simulink model "ActuatorControlLoop"  (R2019a)
settings: Solver=VariableStepAuto  StartTime=0.0  StopTime=10.0  RelTol=1e-3
undefined symbols (not defined in the file or in its folder): Kd, Ki, Kp
settings Model: DataDictionary=HeliSystemDD.sldd  OrderedModelArguments=off  Creator=bpotter  LastModifiedBy=bpotter
settings DataIOCC: ExternalInput=input  LoadExternalInput=on  SaveOutput=off  DSMLogging=off  SaveTime=off  ReturnWorkspaceOutputs=off  ReturnWorkspaceOutputsName=output
settings OptimizationCC: UseDivisionForNetSlopeComputation=on
settings ConfigComp: CovEnable=on  CovScope=ReferencedModels  CovIncludeTopModel=off  CovModelRefEnable=filtered  CovModelRefExcluded=FeedbackDelays,hydraulic_actuator,actuator

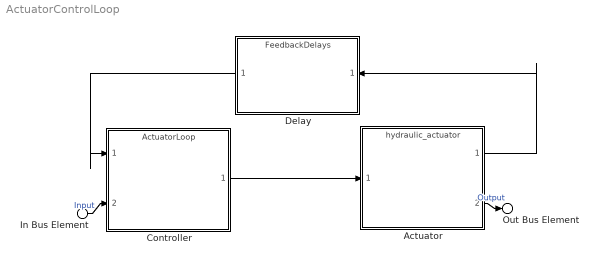
== system ActuatorControlLoop ==
  In Bus Element : Inport  PortName=Command
  Actuator : ModelReference  ModelNameDialog=hydraulic_actuator  SimulationMode=Normal  ModelReferenceVersion=1.109
      settings: PortSchema="{\"entries\":[{\"content\":{\"headerSize\":38,\"margin\":15,\"minimumSpacing\":25,\"sides\":[{\"content\":{\"connectorIds\":[\"In1\"]},\"type\":\"ConnectorPlacement.EquallySpacedRectSide\",\"uuid\":\"01d21f49-5e2a-4880-8609-7c706db9bae6\"},{\"content\":{\"connectorIds\":[\"Out1\",\"Out2\"],\"side\":\"RIGHT\"},\"type\":\"ConnectorPlacement.EquallySpacedRectSide\",\"uuid\":\"8cb49e98-f19c-489e-a3fb-070e8f82a61f\"},{\"content\":{\"connectorIds\":[],\"side\":\"TOP\"},\"type\":\"ConnectorPlacement.EquallySpacedRectSide\",\"uuid\":\"1c2cb19d-116b-4b67-8b19-5c9901225fc1\"}]},\"type\":\"ConnectorPlacement.EquallySpacedConnector\",\"uuid\":\"9f7d65ec-9623-4f05-bd53-df708bb30d55\"}],\"packageUris\":[\"http:\\/\\/schema.mathworks.com\\/mf0\\/Connector\\/19700101\"],\"version\":\"1.0\"}"
  Controller : ModelReference  ModelNameDialog=ActuatorLoop  ParameterArgumentNames=Kp,Kd,Ki  ParameterArgumentValues=0.135,-0.00134,0.00122  UsingDefaultArgumentValue=0,0,0  SimulationMode=Normal  ModelReferenceVersion=1.47
      settings: PortSchema="{\"entries\":[{\"content\":{\"headerSize\":38,\"margin\":15,\"minimumSpacing\":25,\"sides\":[{\"content\":{\"connectorIds\":[\"In1\",\"In2\"]},\"type\":\"ConnectorPlacement.EquallySpacedRectSide\",\"uuid\":\"01d21f49-5e2a-4880-8609-7c706db9bae6\"},{\"content\":{\"connectorIds\":[\"Out1\"],\"side\":\"RIGHT\"},\"type\":\"ConnectorPlacement.EquallySpacedRectSide\",\"uuid\":\"8cb49e98-f19c-489e-a3fb-070e8f82a61f\"},{\"content\":{\"connectorIds\":[],\"side\":\"TOP\"},\"type\":\"ConnectorPlacement.EquallySpacedRectSide\",\"uuid\":\"1c2cb19d-116b-4b67-8b19-5c9901225fc1\"}]},\"type\":\"ConnectorPlacement.EquallySpacedConnector\",\"uuid\":\"9f7d65ec-9623-4f05-bd53-df708bb30d55\"}],\"packageUris\":[\"http:\\/\\/schema.mathworks.com\\/mf0\\/Connector\\/19700101\"],\"version\":\"1.0\"}"
  Delay : ModelReference  ModelNameDialog=FeedbackDelays  SimulationMode=Normal  ModelReferenceVersion=1.165
      settings: PortSchema="{\"entries\":[{\"content\":{\"headerSize\":38,\"margin\":15,\"minimumSpacing\":25,\"sides\":[{\"content\":{\"connectorIds\":[\"Out1\"]},\"type\":\"ConnectorPlacement.EquallySpacedRectSide\",\"uuid\":\"01d21f49-5e2a-4880-8609-7c706db9bae6\"},{\"content\":{\"connectorIds\":[\"In1\"],\"side\":\"RIGHT\"},\"type\":\"ConnectorPlacement.EquallySpacedRectSide\",\"uuid\":\"8cb49e98-f19c-489e-a3fb-070e8f82a61f\"},{\"content\":{\"connectorIds\":[],\"side\":\"TOP\"},\"type\":\"ConnectorPlacement.EquallySpacedRectSide\",\"uuid\":\"1c2cb19d-116b-4b67-8b19-5c9901225fc1\"},{\"content\":{\"connectorIds\":[],\"side\":\"BOTTOM\"},\"type\":\"ConnectorPlacement.EquallySpacedRectSide\",\"uuid\":\"214bcf5f-d005-429b-b513-d0da5e188be9\"}]},\"type\":\"ConnectorPlacement.EquallySpacedConnector\",\"uuid\":\"9f7d65ec-9623-4f05-bd53-df708bb30d55\"}],\"packageUris\":[\"http:\\/\\/schema.mathworks.com\\/mf0\\/Connector\\/19700101\"],\"version\":\"1.0\"}"
  Out Bus Element : Outport  PortName=Position
  wires:
  Controller/1 -> Actuator/1
  Actuator/1 -> Delay/1
  Actuator/2 -> Out Bus Element/1  "Output"
  In Bus Element/1 -> Controller/2  "Input"
  Delay/1 -> Controller/1
